simulink model "problem3"  (R2020b)
settings: Solver=VariableStepAuto  StartTime=0.0  StopTime=10.0  RelTol=1e-3
undefined symbols (not defined in the file): A
libraries: simulink x1
settings Model: Creator=admin  LastModifiedBy=admin

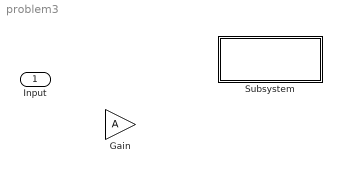
== system problem3 ==
  Input : Inport
  Gain : Gain  Gain=A
  Subsystem : Subsystem

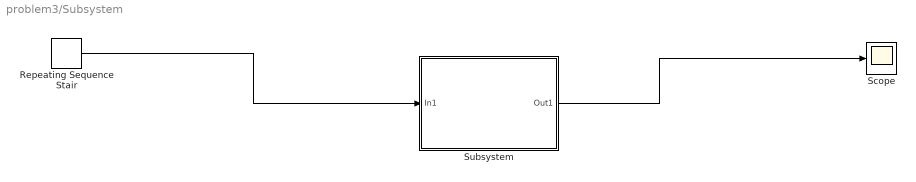
== system problem3/Subsystem ==
  Repeating Sequence Stair : simulink/Sources/Repeating Sequence Stair  OutValues=[1 0 0 0 1]  tsamp=-1  OutMin=[]  OutMax=[]  OutDataTypeStr=double  OutputDataTypeScalingMode=double  OutDataType=fixdt(0,8)  ConRadixGroup=Best Precision: Vector-wise  OutScaling=2^-12
  Scope : Scope
  Subsystem : Subsystem
  wires:
  Repeating Sequence Stair/1 -> Subsystem/1(In1)
  Subsystem/1(Out1) -> Scope/1

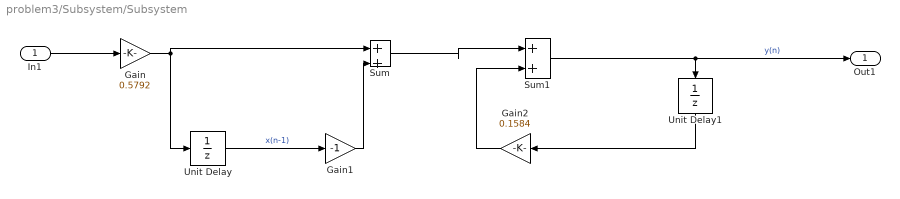
== system problem3/Subsystem/Subsystem ==
  In1 : Inport
  Gain : Gain  Gain=0.5792
  Gain1 : Gain  Gain=-1
  Gain2 : Gain  Gain=0.1584
  Sum : Sum  Inputs=|++
  Sum1 : Sum  Inputs=|++
  Unit Delay : UnitDelay  SampleTime=-1  HasFrameUpgradeWarning=on
  Unit Delay1 : UnitDelay  SampleTime=-1  HasFrameUpgradeWarning=on
  Out1 : Outport
  wires:
  Gain/1 -> Sum/1, Unit Delay/1
  In1/1 -> Gain/1
  Sum1/1 -> Out1/1, Unit Delay1/1  "y(n)"
  Sum/1 -> Sum1/1
  Unit Delay/1 -> Gain1/1  "x(n-1)"
  Gain1/1 -> Sum/2
  Gain2/1 -> Sum1/2
  Unit Delay1/1 -> Gain2/1
